simulink model "gm_CustArch_vnl"  (R2020a)
settings: Solver=FixedStepDiscrete  StartTime=0.0  StopTime=7e4  RelTol=1e-3
libraries: simulink x176, hdlsllib x104, hdlmdlgenlib x2, dsparch4 x1
(part 3 of 4)

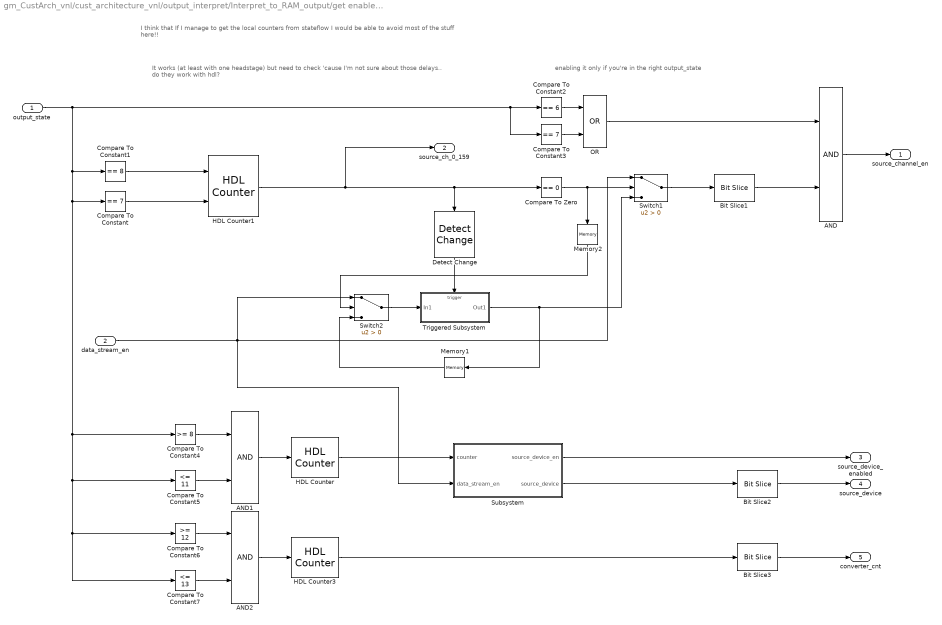
== system gm_CustArch_vnl/cust_architecture_vnl/output_interpret/Interpret_to_RAM_output/get enabled timings  ==
  note: It works (at least with one headstage) but need to check 'cause I'm not sure about those delays.. do they work with hdl?
  note: enabling it only if you're in the right output_state
  note: I think that If I manage to get the local counters from stateflow I would be able to avoid most of the stuff here!!
  output_state : Inport
  data_stream_en : Inport  Port=2
  AND : Logic  IconShape=distinctive  AllPortsSameDT=off  OutDataTypeStr=boolean
  AND1 : Logic  IconShape=distinctive  AllPortsSameDT=off  OutDataTypeStr=boolean
  AND2 : Logic  IconShape=distinctive  AllPortsSameDT=off  OutDataTypeStr=boolean
  Bit Slice1 : hdlsllib/Logic and Bit Operations/Bit Slice  lidx=0  ridx=0
      settings: SourceProductBaseCode=SL
  Bit Slice2 : hdlsllib/Logic and Bit Operations/Bit Slice  lidx=2  ridx=0
      settings: SourceProductBaseCode=SL
  Bit Slice3 : hdlsllib/Logic and Bit Operations/Bit Slice  lidx=2  ridx=0
      settings: SourceProductBaseCode=SL
  Compare To Constant : simulink/Logic and Bit Operations/Compare To Constant  relop===  const=7  OutDataTypeStr=boolean
  Compare To Constant1 : simulink/Logic and Bit Operations/Compare To Constant  relop===  const=8  OutDataTypeStr=boolean
  Compare To Constant2 : simulink/Logic and Bit Operations/Compare To Constant  relop===  const=6  OutDataTypeStr=boolean
  Compare To Constant3 : simulink/Logic and Bit Operations/Compare To Constant  relop===  const=7  OutDataTypeStr=boolean
  Compare To Constant4 : simulink/Logic and Bit Operations/Compare To Constant  relop=>=  const=8  OutDataTypeStr=boolean
  Compare To Constant5 : simulink/Logic and Bit Operations/Compare To Constant  relop=<=  const=11  OutDataTypeStr=boolean
  Compare To Constant6 : simulink/Logic and Bit Operations/Compare To Constant  relop=>=  const=12  OutDataTypeStr=boolean
  Compare To Constant7 : simulink/Logic and Bit Operations/Compare To Constant  relop=<=  const=13  OutDataTypeStr=boolean
  Compare To Zero : simulink/Logic and Bit Operations/Compare To Zero  relop===  OutDataTypeStr=boolean
  Detect Change : simulink/Logic and Bit Operations/Detect Change  vinit=0  OutDataTypeStr=boolean
  HDL Counter : hdlsllib/Sources/HDL Counter  CountType=Count limited  CountInit=0  CountStep=1  CountMax=7  CountFromType=Specify  CountFrom=0  CountResetPort=off  CountLoadPort=off  CountEnbPort=on  CountDirPort=off  CountDataType=Unsigned  CountWordLen=8  CountFracLen=0  CountSampTime=1
  HDL Counter1 : hdlsllib/Sources/HDL Counter  CountType=Count limited  CountInit=0  CountStep=1  CountMax=159  CountFromType=Specify  CountFrom=0  CountResetPort=on  CountLoadPort=off  CountEnbPort=on  CountDirPort=off  CountDataType=Unsigned  CountWordLen=8  CountFracLen=0  CountSampTime=1
  HDL Counter3 : hdlsllib/Sources/HDL Counter  CountType=Count limited  CountInit=0  CountStep=1  CountMax=7  CountFromType=Specify  CountFrom=0  CountResetPort=off  CountLoadPort=off  CountEnbPort=on  CountDirPort=off  CountDataType=Unsigned  CountWordLen=8  CountFracLen=0  CountSampTime=1
  Memory1 : Memory  InheritSampleTime=on
  Memory2 : Memory  InheritSampleTime=on
  OR : Logic  Operator=OR  IconShape=distinctive  AllPortsSameDT=off  OutDataTypeStr=boolean
  Subsystem : Subsystem
  Switch1 : Switch  Criteria=u2 > Threshold
  Switch2 : Switch  Criteria=u2 > Threshold
  Triggered Subsystem : Subsystem  TreatAsAtomicUnit=on
  source_channel_en : Outport  VectorParamsAs1DForOutWhenUnconnected=off
  source_ch_0_159 : Outport  Port=2  OutMin=0  OutMax=159  OutDataTypeStr=uint8  VectorParamsAs1DForOutWhenUnconnected=off  LockScale=on
  source_device_enabled : Outport  Port=3  VectorParamsAs1DForOutWhenUnconnected=off
  source_device : Outport  Port=4  VectorParamsAs1DForOutWhenUnconnected=off
  converter_cnt : Outport  Port=5  VectorParamsAs1DForOutWhenUnconnected=off
  wires:
  Compare To Constant/1 -> HDL Counter1/2
  Compare To Constant1/1 -> HDL Counter1/1
  HDL Counter3/1 -> Bit Slice3/1
  AND2/1 -> HDL Counter3/1
  Compare To Constant7/1 -> AND2/2
  output_state/1 -> Compare To Constant2/1, Compare To Constant3/1, Compare To Constant4/1, Compare To Constant5/1, Compare To Constant7/1, Compare To Constant6/1, Compare To Constant/1, Compare To Constant1/1
  Bit Slice3/1 -> converter_cnt/1
  Compare To Constant6/1 -> AND2/1
  data_stream_en/1 -> Switch2/1, Subsystem/2(data_stream_en), Switch1/1
  Subsystem/2(source_device) -> Bit Slice2/1
  HDL Counter/1 -> Subsystem/1("counter ")
  AND1/1 -> HDL Counter/1
  Bit Slice2/1 -> source_device/1
  Subsystem/1(source_device_en) -> source_device_enabled/1
  Compare To Constant5/1 -> AND1/2
  Compare To Constant4/1 -> AND1/1
  Bit Slice1/1 -> AND/2
  Switch1/1 -> Bit Slice1/1
  AND/1 -> source_channel_en/1
  OR/1 -> AND/1
  Compare To Constant2/1 -> OR/1
  Compare To Constant3/1 -> OR/2
  Memory2/1 -> Switch2/2
  Compare To Zero/1 -> Memory2/1, Switch1/2
  Switch2/1 -> Triggered Subsystem/1(In1)
  Memory1/1 -> Switch2/3
  Triggered Subsystem/1(Out1) -> Switch1/3, Memory1/1
  Detect Change/1 -> Triggered Subsystem/Trigger
  HDL Counter1/1 -> source_ch_0_159/1, Compare To Zero/1, Detect Change/1

== system gm_CustArch_vnl/cust_architecture_vnl/process_and_retrieve/80-120Hz IIR/Filter ==
  In : Inport
  Input Quantizer : DataTypeConversion  OutDataTypeStr=fixdt(1,16,15)  RndMeth=Round  SaturateOnIntegerOverflow=on
  filter : dsparch4/Biquad Filter  FilterSource=Dialog parameters  CoeffSource=Specify via dialog  FilterObject=BQF  IIRFiltStruct=Direct form II  BiQuadCoeffs=[1 0 -1 1 -1.99840418478311443 0.999052538203115237;1 0 -1 1 -1.99911154185162543 0.999384811657715533;1 0 -1 1 -1.99656292392472823 0.997202711747327109;1 0 -1 1 -1.99788402546849486 0.998160528507833211;1 0 -1 1 -1.99485713531997422 0.995480866402445264;1 0 -1 1 -1.99667039725885465 0.996953603258886489;1 0 -1 1 -1.99336016454168963 0.993961190148174412;1 0 -1 1 -1.99548437511557175 0.995777884172216132;1 0 -1 1 -1.992132714994862 0.992705563421812376;1 0 -1 1 -1.99434459502704264 0.994652174705462522;1 0 -1 1 -1.99121885243658769 0.991759490866001236;1 0 -1 1 -1.99327645890654415 0.99360203837599903;1 0 -1 1 -1.99064291385656711 0.991148910200749356;1 0 -1 1 -1.99231340829021986 0.992661008227186614;1 0 -1 1 -1.99040799304795324 0.990878552519449007;1 0 -1 1 -1.99149697231721445 0.991870551163973602;1 0 -1 1 -1.990496738771526 0.990932601430571158;1 0 -1 1 -1.99087486526267554 0.991278074310207646]  ScaleValues=[0.0044824738599215392;0.0044824738599215392;0.00447903005734254407;0.00447903005734254407;0.00447575140857445122;0.00447575140857445122;0.00447273615619287867;0.00447273615619287867;0.004470074082001705;0.004470074082001705;0.004467844000312143;0.004467844000312143;0.00446611161073571031;0.00446611161073571031;0.00446492774650666859;0.00446492774650666859;0.00446432704310449711;0.00446432704310449711;1]  IC=0  ICnum=0  ICden=0  a0Flag=Warning  optimizeScaleValues=on  ScaleValueMode=Specify via input port (g)  InputProcessing=Columns as channels (frame based)  roundingMode=Convergent  overflowMode=off  stageInputMode=Binary point scaling  stageInputWordLength=16  stageInputFracLength=17  stageOutputMode=Binary point scaling  stageOutputWordLength=16  stageOutputFracLength=11  firstCoeffMode=Binary point scaling  firstCoeffWordLength=16  firstCoeffFracLength=14  scaleValueFracLength=22  prodOutputMode=Binary point scaling  prodOutputWordLength=32  prodOutputFracLength=29  denProdOutputFracLength=29  accumMode=Binary point scaling  accumWordLength=40  accumFracLength=29  denAccumFracLength=29  memoryMode=Binary point scaling  memoryWordLength=16  memoryFracLength=15  secondMemoryFracLength=15  outputMode=Binary point scaling  outputWordLength=16  outputFracLength=11
  Out : Outport
  wires:
  filter/1 -> Out/1
  Input Quantizer/1 -> filter/1
  In/1 -> Input Quantizer/1

== system gm_CustArch_vnl/cust_architecture_vnl/process_and_retrieve/one_pole_IIR/Filter1 ==
  Input : Inport  OutDataTypeStr=fixdt(1,16,0)
  Input1 : Inport  Port=2
  SumA21 : Sum  Inputs=|+-  OutDataTypeStr=fixdt(1,16,-5)  RndMeth=Nearest  SaturateOnIntegerOverflow=on
  SumB21 : Sum  Inputs=|+-  OutDataTypeStr=fixdt(1,16,-1)  RndMeth=Nearest  SaturateOnIntegerOverflow=on
  a(2)(1) : Gain  Gain=-0.939062505817492399  ParamDataTypeStr=fixdt(1,16,15)  OutDataTypeStr=fixdt(1,16,-4)  RndMeth=Nearest  SaturateOnIntegerOverflow=on
  s(1) : Gain  Gain=0.969531252908746199  ParamDataTypeStr=fixdt(0,16,16)  OutDataTypeStr=fixdt(1,16,0)  RndMeth=Nearest  SaturateOnIntegerOverflow=on
  Output : Outport  VectorParamsAs1DForOutWhenUnconnected=off
  Output1 : Outport  Port=2  VectorParamsAs1DForOutWhenUnconnected=off
  wires:
  Input1/1 -> SumB21/2, a(2)(1)/1
  a(2)(1)/1 -> SumA21/2
  SumB21/1 -> Output/1
  SumA21/1 -> SumB21/1, Output1/1
  s(1)/1 -> SumA21/1
  Input/1 -> s(1)/1

== system gm_CustArch_vnl/cust_architecture/input_interpret_store_retrieve/Interpret_to_RAM_input/interpret data/condition to count DAC or ADC  ==
  fifo_write_to : Inport  OutDataTypeStr=boolean  PortDimensions=1  SampleTime=1
  input_state : Inport  Port=2  OutDataTypeStr=uint8  PortDimensions=1  SampleTime=1
  AND : Logic  AllPortsSameDT=off  OutDataTypeStr=boolean  SampleTime=1
  OR : Logic  Operator=OR  AllPortsSameDT=off  OutDataTypeStr=boolean  SampleTime=1
  is state_ADC : simulink/Logic and Bit Operations/Compare To Constant  relop===  const="fi(0,0,8,0,\"hex\",\"0d\")"  OutDataTypeStr=boolean
  is state_DAC : simulink/Logic and Bit Operations/Compare To Constant  relop===  const="fi(0,0,8,0,\"hex\",\"0c\")"  OutDataTypeStr=boolean
  Out1 : Outport  VectorParamsAs1DForOutWhenUnconnected=off
  wires:
  is state_DAC/1 -> OR/1
  is state_ADC/1 -> OR/2
  OR/1 -> AND/2
  AND/1 -> Out1/1
  input_state/1 -> is state_ADC/1, is state_DAC/1
  fifo_write_to/1 -> AND/1

== system gm_CustArch_vnl/cust_architecture/input_interpret_store_retrieve/Interpret_to_RAM_input/interpret data/get_sources ==
  note: 0-159 --> 20(16+4)x8
  note: chiedere cose
  note: identifichi chip che stai leggendo
  note: se next è tutto di zeri allora siamo a un nuovo channel (0-19)
  FIFO_write_to : Inport  OutDataTypeStr=boolean  PortDimensions=1  SampleTime=1
  InputState : Inport  Port=2  OutDataTypeStr=uint8  PortDimensions=1  SampleTime=1
  data_stream_enable : Inport  Port=3  OutDataTypeStr=uint8  PortDimensions=1  SampleTime=1
  AND{,1..3} (4 alike) : Logic  AllPortsSameDT=off  OutDataTypeStr=boolean  SampleTime=1
  Compare To Constant1 : simulink/Logic and Bit Operations/Compare To Constant  relop===  const="fi(0,0,8,0,\"hex\",\"00\")"  OutDataTypeStr=boolean
  Compare To Constant2 : simulink/Logic and Bit Operations/Compare To Constant  relop===  const="fi(0,0,8,0,\"hex\",\"0d\")"  OutDataTypeStr=boolean
  Compare To Constant3 : simulink/Logic and Bit Operations/Compare To Constant  relop===  const="fi(0,0,8,0,\"hex\",\"06\")"  OutDataTypeStr=boolean
  Compare To Constant4 : simulink/Logic and Bit Operations/Compare To Constant  relop=>=  const="fi(0,0,8,0,\"hex\",\"08\")"  OutDataTypeStr=boolean
  Compare To Constant5 : simulink/Logic and Bit Operations/Compare To Constant  relop===  const="fi(0,0,8,0,\"hex\",\"00\")"  OutDataTypeStr=boolean
  Compare To Constant6 : simulink/Logic and Bit Operations/Compare To Constant  relop=<=  const="fi(0,0,8,0,\"hex\",\"0b\")"  OutDataTypeStr=boolean
  HDL Counter : hdlsllib/Sources/HDL Counter  CountType=Count limited  CountInit=double(0)  CountStep=double(1)  CountMax=double(20)  CountFromType=Initial value  CountFrom=double(0)  CountResetPort=on  CountLoadPort=off  CountEnbPort=on  CountDirPort=off  CountDataType=Unsigned  CountWordLen=8  CountFracLen=0  CountSampTime=1
  Memory : UnitDelay  InitialCondition=double(0)  SampleTime=1
  Memory1 : UnitDelay  InitialCondition=double(0)  SampleTime=1
  Memory2 : UnitDelay  InitialCondition=double(0)  SampleTime=1
  OR : Logic  Operator=OR  AllPortsSameDT=off  OutDataTypeStr=boolean  SampleTime=1
  Subsystem : Subsystem
  Switch : Switch  Criteria=u2 > Threshold  Threshold=double(0)  OutDataTypeStr=uint8  SampleTime=1
  Switch1 : Switch  Criteria=u2 > Threshold  Threshold=double(0)  OutDataTypeStr=uint8  SampleTime=1
  Triggered Subsystem : Subsystem
  find_first_one_pos : Subsystem
  position_to_bitmask : Subsystem
  source_device : Outport  VectorParamsAs1DForOutWhenUnconnected=off
  dev_out_channel_0_19 : Outport  Port=2  VectorParamsAs1DForOutWhenUnconnected=off
  source_channel : Outport  Port=3  VectorParamsAs1DForOutWhenUnconnected=off
  bitmasked==0 : Outport  Port=4  VectorParamsAs1DForOutWhenUnconnected=off
  wires:
  position_to_bitmask/1(bit_masked) -> Memory/1, Compare To Constant5/1
  find_first_one_pos/1(first_one_pos) -> Triggered Subsystem/1(In1), position_to_bitmask/2(first_one_pos)
  Triggered Subsystem/1(Out1) -> Subsystem/1(source_device), source_device/1
  Switch1/1 -> Switch/3
  Switch/1 -> find_first_one_pos/1(In1), position_to_bitmask/1(curr_channel_rollmap)
  Subsystem/1(source_channel_0_159) -> source_channel/1
  OR/1 -> AND/2
  Memory2/1 -> AND3/2
  Memory1/1 -> AND3/1, Switch1/2
  Memory/1 -> Switch1/3
  HDL Counter/1 -> Subsystem/2(dev_output), dev_out_channel_0_19/1
  Compare To Constant6/1 -> AND1/2
  Compare To Constant5/1 -> Memory1/1, AND2/2
  Compare To Constant4/1 -> AND1/1
  Compare To Constant3/1 -> OR/1
  Compare To Constant2/1 -> HDL Counter/1
  Compare To Constant1/1 -> Switch/2
  AND3/1 -> HDL Counter/2
  AND2/1 -> bitmasked==0/1
  AND1/1 -> OR/2
  AND/1 -> find_first_one_pos/Enable, position_to_bitmask/Enable, Subsystem/Enable, Triggered Subsystem/Enable, Memory2/1, AND2/1
  data_stream_enable/1 -> Switch/1, Switch1/1
  InputState/1 -> Compare To Constant1/1, Compare To Constant2/1, Compare To Constant3/1, Compare To Constant4/1, Compare To Constant6/1
  FIFO_write_to/1 -> AND/1

== system gm_CustArch_vnl/cust_architecture/output_interpret/Interpret_to_RAM_output/get enabled timings /Subsystem ==
  "counter " : Inport  OutDataTypeStr=uint8  PortDimensions=1  SampleTime=1
  data_stream_en : Inport  Port=2  OutDataTypeStr=uint8  PortDimensions=1  SampleTime=1
  Bit Rotate : hdlsllib/Logic and Bit Operations/Bit Rotate  mode=Rotate Right  N=double(1)
      settings: SourceProductBaseCode=SL
  Bit Rotate1 : hdlsllib/Logic and Bit Operations/Bit Rotate  mode=Rotate Right  N=double(2)
      settings: SourceProductBaseCode=SL
  Bit Rotate2 : hdlsllib/Logic and Bit Operations/Bit Rotate  mode=Rotate Right  N=double(3)
      settings: SourceProductBaseCode=SL
  Bit Rotate3 : hdlsllib/Logic and Bit Operations/Bit Rotate  mode=Rotate Right  N=double(4)
      settings: SourceProductBaseCode=SL
  Bit Rotate4 : hdlsllib/Logic and Bit Operations/Bit Rotate  mode=Rotate Right  N=double(5)
      settings: SourceProductBaseCode=SL
  Bit Rotate5 : hdlsllib/Logic and Bit Operations/Bit Rotate  mode=Rotate Right  N=double(6)
      settings: SourceProductBaseCode=SL
  Bit Rotate6 : hdlsllib/Logic and Bit Operations/Bit Rotate  mode=Rotate Right  N=double(7)
      settings: SourceProductBaseCode=SL
  Bit Slice : hdlsllib/Logic and Bit Operations/Bit Slice  lidx=double(0)  ridx=double(0)
      settings: SourceProductBaseCode=SL
  Compare To Constant : simulink/Logic and Bit Operations/Compare To Constant  relop===  const="fi(0,0,8,0,\"hex\",\"00\")"  OutDataTypeStr=boolean
  Compare To Constant1 : simulink/Logic and Bit Operations/Compare To Constant  relop===  const="fi(0,0,8,0,\"hex\",\"01\")"  OutDataTypeStr=boolean
  Compare To Constant2 : simulink/Logic and Bit Operations/Compare To Constant  relop===  const="fi(0,0,8,0,\"hex\",\"02\")"  OutDataTypeStr=boolean
  Compare To Constant3 : simulink/Logic and Bit Operations/Compare To Constant  relop===  const="fi(0,0,8,0,\"hex\",\"03\")"  OutDataTypeStr=boolean
  Compare To Constant4 : simulink/Logic and Bit Operations/Compare To Constant  relop===  const="fi(0,0,8,0,\"hex\",\"04\")"  OutDataTypeStr=boolean
  Compare To Constant5 : simulink/Logic and Bit Operations/Compare To Constant  relop===  const="fi(0,0,8,0,\"hex\",\"05\")"  OutDataTypeStr=boolean
  Compare To Constant6 : simulink/Logic and Bit Operations/Compare To Constant  relop===  const="fi(0,0,8,0,\"hex\",\"06\")"  OutDataTypeStr=boolean
  Compare To Constant7 : simulink/Logic and Bit Operations/Compare To Constant  relop===  const="fi(0,0,8,0,\"hex\",\"07\")"  OutDataTypeStr=boolean
  Constant : Constant  Value=0  OutDataTypeStr=uint8  SampleTime=1
  Switch{,1..7} (8 alike) : Switch  Criteria=u2 > Threshold  Threshold=double(0)  OutDataTypeStr=uint8  SampleTime=1
  source_device_en : Outport  VectorParamsAs1DForOutWhenUnconnected=off
  source_device : Outport  Port=2  VectorParamsAs1DForOutWhenUnconnected=off
  wires:
  Switch7/1 -> Switch6/3
  Switch6/1 -> Switch5/3
  Switch5/1 -> Switch4/3
  Switch4/1 -> Switch3/3
  Switch3/1 -> Switch2/3
  Switch2/1 -> Switch1/3
  Switch1/1 -> Switch/3
  Switch/1 -> Bit Slice/1
  Constant/1 -> Switch7/3
  Compare To Constant7/1 -> Switch7/2
  Compare To Constant6/1 -> Switch6/2
  Compare To Constant5/1 -> Switch5/2
  Compare To Constant4/1 -> Switch4/2
  Compare To Constant3/1 -> Switch3/2
  Compare To Constant2/1 -> Switch2/2
  Compare To Constant1/1 -> Switch1/2
  Compare To Constant/1 -> Switch/2
  Bit Slice/1 -> source_device_en/1
  Bit Rotate6/1 -> Switch7/1
  Bit Rotate5/1 -> Switch6/1
  Bit Rotate4/1 -> Switch5/1
  Bit Rotate3/1 -> Switch4/1
  Bit Rotate2/1 -> Switch3/1
  Bit Rotate1/1 -> Switch2/1
  Bit Rotate/1 -> Switch1/1
  data_stream_en/1 -> Bit Rotate/1, Bit Rotate1/1, Bit Rotate2/1, Bit Rotate3/1, Bit Rotate4/1, Bit Rotate5/1, Bit Rotate6/1, Switch/1
  "counter "/1 -> source_device/1, Compare To Constant/1, Compare To Constant1/1, Compare To Constant2/1, Compare To Constant3/1, Compare To Constant4/1, Compare To Constant5/1, Compare To Constant6/1, Compare To Constant7/1

== system gm_CustArch_vnl/cust_architecture/output_interpret/Interpret_to_RAM_output/get enabled timings /Triggered Subsystem ==
  In1 : Inport  OutDataTypeStr=uint8  PortDimensions=1
  Trigger : TriggerPort  VariantControl=(inherit)  PortDimensions=1  OutDataTypeStr=boolean
  Bit Rotate : hdlsllib/Logic and Bit Operations/Bit Rotate  mode=Rotate Right  N=double(1)
      settings: SourceProductBaseCode=SL
  Out1 : Outport  InitialOutput=0  VectorParamsAs1DForOutWhenUnconnected=off
  wires:
  Bit Rotate/1 -> Out1/1
  In1/1 -> Bit Rotate/1

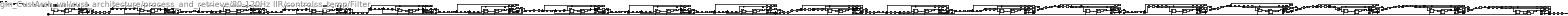
== system gm_CustArch_vnl/cust_architecture/process_and_retrieve/80-120Hz IIR/controlss_temp/Filter ==
  In : Inport  OutDataTypeStr=fixdt(1, 16, 15)  PortDimensions=1  SampleTime=1
  Trigger_emulated : Inport  Port=2  OutDataTypeStr=boolean  SampleTime=1
  Input Quantizer : DataTypeConversion  OutDataTypeStr=fixdt(1, 16, 15)  RndMeth=Round  SampleTime=1  SaturateOnIntegerOverflow=on
  Sub{,1..35} (36 alike) : Sum  Inputs=+-  OutDataTypeStr=fixdt(1, 41, 29)  RndMeth=Convergent  SampleTime=1
  adder{,1..17} (18 alike) : Sum  OutDataTypeStr=fixdt(1, 40, 29)  RndMeth=Convergent  SampleTime=1
  const : Constant  Value=0.0044825077056884765625  OutDataTypeStr=fixdt(1, 16, 22)  SampleTime=1
  const1 : Constant  Value=-1.9984130859375  OutDataTypeStr=fixdt(1, 16, 14)  SampleTime=1
  const10 : Constant  Value=-1.99786376953125  OutDataTypeStr=fixdt(1, 16, 14)  SampleTime=1
  const11 : Constant  Value=0.9981689453125  OutDataTypeStr=fixdt(1, 16, 14)  SampleTime=1
  const12 : Constant  Value=0.0044758319854736328125  OutDataTypeStr=fixdt(1, 16, 22)  SampleTime=1
  const13 : Constant  Value=-1.994873046875  OutDataTypeStr=fixdt(1, 16, 14)  SampleTime=1
  const14 : Constant  Value=0.9954833984375  OutDataTypeStr=fixdt(1, 16, 14)  SampleTime=1
  const15 : Constant  Value=0.0044758319854736328125  OutDataTypeStr=fixdt(1, 16, 22)  SampleTime=1
  const16 : Constant  Value=-1.99664306640625  OutDataTypeStr=fixdt(1, 16, 14)  SampleTime=1
  const17 : Constant  Value=0.9969482421875  OutDataTypeStr=fixdt(1, 16, 14)  SampleTime=1
  const18 : Constant  Value=0.0044727325439453125  OutDataTypeStr=fixdt(1, 16, 22)  SampleTime=1
  const19 : Constant  Value=-1.99334716796875  OutDataTypeStr=fixdt(1, 16, 14)  SampleTime=1
  const2 : Constant  Value=0.9990234375  OutDataTypeStr=fixdt(1, 16, 14)  SampleTime=1
  const20 : Constant  Value=0.99395751953125  OutDataTypeStr=fixdt(1, 16, 14)  SampleTime=1
  const21 : Constant  Value=0.0044727325439453125  OutDataTypeStr=fixdt(1, 16, 22)  SampleTime=1
  const22 : Constant  Value=-1.9954833984375  OutDataTypeStr=fixdt(1, 16, 14)  SampleTime=1
  const23 : Constant  Value=0.99578857421875  OutDataTypeStr=fixdt(1, 16, 14)  SampleTime=1
  const24 : Constant  Value=0.0044701099395751953125  OutDataTypeStr=fixdt(1, 16, 22)  SampleTime=1
  const25 : Constant  Value=-1.99212646484375  OutDataTypeStr=fixdt(1, 16, 14)  SampleTime=1
  const26 : Constant  Value=0.99267578125  OutDataTypeStr=fixdt(1, 16, 14)  SampleTime=1
  const27 : Constant  Value=0.0044701099395751953125  OutDataTypeStr=fixdt(1, 16, 22)  SampleTime=1
  const28 : Constant  Value=-1.99432373046875  OutDataTypeStr=fixdt(1, 16, 14)  SampleTime=1
  const29 : Constant  Value=0.99462890625  OutDataTypeStr=fixdt(1, 16, 14)  SampleTime=1
  const3 : Constant  Value=0.0044825077056884765625  OutDataTypeStr=fixdt(1, 16, 22)  SampleTime=1
  const30 : Constant  Value=0.0044677257537841796875  OutDataTypeStr=fixdt(1, 16, 22)  SampleTime=1
  const31 : Constant  Value=-1.9912109375  OutDataTypeStr=fixdt(1, 16, 14)  SampleTime=1
  const32 : Constant  Value=0.99176025390625  OutDataTypeStr=fixdt(1, 16, 14)  SampleTime=1
  const33 : Constant  Value=0.0044677257537841796875  OutDataTypeStr=fixdt(1, 16, 22)  SampleTime=1
  const34 : Constant  Value=-1.9932861328125  OutDataTypeStr=fixdt(1, 16, 14)  SampleTime=1
  const35 : Constant  Value=0.99359130859375  OutDataTypeStr=fixdt(1, 16, 14)  SampleTime=1
  const36 : Constant  Value=0.00446605682373046875  OutDataTypeStr=fixdt(1, 16, 22)  SampleTime=1
  const37 : Constant  Value=-1.99066162109375  OutDataTypeStr=fixdt(1, 16, 14)  SampleTime=1
  const38 : Constant  Value=0.99114990234375  OutDataTypeStr=fixdt(1, 16, 14)  SampleTime=1
  const39 : Constant  Value=0.00446605682373046875  OutDataTypeStr=fixdt(1, 16, 22)  SampleTime=1
  const4 : Constant  Value=-1.99908447265625  OutDataTypeStr=fixdt(1, 16, 14)  SampleTime=1
  const40 : Constant  Value=-1.9923095703125  OutDataTypeStr=fixdt(1, 16, 14)  SampleTime=1
  const41 : Constant  Value=0.99267578125  OutDataTypeStr=fixdt(1, 16, 14)  SampleTime=1
  const42 : Constant  Value=0.0044648647308349609375  OutDataTypeStr=fixdt(1, 16, 22)  SampleTime=1
  const43 : Constant  Value=-1.99041748046875  OutDataTypeStr=fixdt(1, 16, 14)  SampleTime=1
  const44 : Constant  Value=0.99090576171875  OutDataTypeStr=fixdt(1, 16, 14)  SampleTime=1
  const45 : Constant  Value=0.0044648647308349609375  OutDataTypeStr=fixdt(1, 16, 22)  SampleTime=1
  const46 : Constant  Value=-1.99151611328125  OutDataTypeStr=fixdt(1, 16, 14)  SampleTime=1
  const47 : Constant  Value=0.99188232421875  OutDataTypeStr=fixdt(1, 16, 14)  SampleTime=1
  const48 : Constant  Value=0.0044643878936767578125  OutDataTypeStr=fixdt(1, 16, 22)  SampleTime=1
  const49 : Constant  Value=-1.990478515625  OutDataTypeStr=fixdt(1, 16, 14)  SampleTime=1
  const5 : Constant  Value=0.9993896484375  OutDataTypeStr=fixdt(1, 16, 14)  SampleTime=1
  const50 : Constant  Value=0.99090576171875  OutDataTypeStr=fixdt(1, 16, 14)  SampleTime=1
  const51 : Constant  Value=0.0044643878936767578125  OutDataTypeStr=fixdt(1, 16, 22)  SampleTime=1
  const52 : Constant  Value=-1.9908447265625  OutDataTypeStr=fixdt(1, 16, 14)  SampleTime=1
  const53 : Constant  Value=0.99127197265625  OutDataTypeStr=fixdt(1, 16, 14)  SampleTime=1
  const6 : Constant  Value=0.004478931427001953125  OutDataTypeStr=fixdt(1, 16, 22)  SampleTime=1
  const7 : Constant  Value=-1.99658203125  OutDataTypeStr=fixdt(1, 16, 14)  SampleTime=1
  const8 : Constant  Value=0.9971923828125  OutDataTypeStr=fixdt(1, 16, 14)  SampleTime=1
  const9 : Constant  Value=0.004478931427001953125  OutDataTypeStr=fixdt(1, 16, 22)  SampleTime=1
  delay_process_section10_tap0 : Subsystem
      settings: MinAlgLoopOccurrences=on
  delay_process_section10_tap1 : Subsystem
      settings: MinAlgLoopOccurrences=on
  delay_process_section11_tap0 : Subsystem
      settings: MinAlgLoopOccurrences=on
  delay_process_section11_tap1 : Subsystem
      settings: MinAlgLoopOccurrences=on
  delay_process_section12_tap0 : Subsystem
      settings: MinAlgLoopOccurrences=on
  delay_process_section12_tap1 : Subsystem
      settings: MinAlgLoopOccurrences=on
  delay_process_section13_tap0 : Subsystem
      settings: MinAlgLoopOccurrences=on
  delay_process_section13_tap1 : Subsystem
      settings: MinAlgLoopOccurrences=on
  delay_process_section14_tap0 : Subsystem
      settings: MinAlgLoopOccurrences=on
  delay_process_section14_tap1 : Subsystem
      settings: MinAlgLoopOccurrences=on
  delay_process_section15_tap0 : Subsystem
      settings: MinAlgLoopOccurrences=on
  delay_process_section15_tap1 : Subsystem
      settings: MinAlgLoopOccurrences=on
  delay_process_section16_tap0 : Subsystem
      settings: MinAlgLoopOccurrences=on
  delay_process_section16_tap1 : Subsystem
      settings: MinAlgLoopOccurrences=on
  delay_process_section17_tap0 : Subsystem
      settings: MinAlgLoopOccurrences=on
  delay_process_section17_tap1 : Subsystem
      settings: MinAlgLoopOccurrences=on
  delay_process_section18_tap0 : Subsystem
      settings: MinAlgLoopOccurrences=on
  delay_process_section18_tap1 : Subsystem
      settings: MinAlgLoopOccurrences=on
  delay_process_section1_tap0 : Subsystem
      settings: MinAlgLoopOccurrences=on
  delay_process_section1_tap1 : Subsystem
      settings: MinAlgLoopOccurrences=on
  delay_process_section2_tap0 : Subsystem
      settings: MinAlgLoopOccurrences=on
  delay_process_section2_tap1 : Subsystem
      settings: MinAlgLoopOccurrences=on
  delay_process_section3_tap0 : Subsystem
      settings: MinAlgLoopOccurrences=on
  delay_process_section3_tap1 : Subsystem
      settings: MinAlgLoopOccurrences=on
  delay_process_section4_tap0 : Subsystem
      settings: MinAlgLoopOccurrences=on
  delay_process_section4_tap1 : Subsystem
      settings: MinAlgLoopOccurrences=on
  delay_process_section5_tap0 : Subsystem
      settings: MinAlgLoopOccurrences=on
  delay_process_section5_tap1 : Subsystem
      settings: MinAlgLoopOccurrences=on
  delay_process_section6_tap0 : Subsystem
      settings: MinAlgLoopOccurrences=on
  delay_process_section6_tap1 : Subsystem
      settings: MinAlgLoopOccurrences=on
  delay_process_section7_tap0 : Subsystem
      settings: MinAlgLoopOccurrences=on
  delay_process_section7_tap1 : Subsystem
      settings: MinAlgLoopOccurrences=on
  delay_process_section8_tap0 : Subsystem
      settings: MinAlgLoopOccurrences=on
  delay_process_section8_tap1 : Subsystem
      settings: MinAlgLoopOccurrences=on
  delay_process_section9_tap0 : Subsystem
      settings: MinAlgLoopOccurrences=on
  delay_process_section9_tap1 : Subsystem
      settings: MinAlgLoopOccurrences=on
  dtc{,11,22,33,44,55,66,77,88,99,110,121,132,143,154,165,176,187} (18 alike) : DataTypeConversion  OutDataTypeStr=fixdt(1, 16, 17)  RndMeth=Convergent  SampleTime=1
  dtc{1,12,23,34,45,56,67,78,89,100,111,122,133,144,155,166,177,188} (18 alike) : DataTypeConversion  OutDataTypeStr=fixdt(1, 16, 15)  RndMeth=Convergent  SampleTime=1
  dtc{10,21,32,43,54,65,76,87,98,109,120,131,142,153,164,175,186,197} (18 alike) : DataTypeConversion  OutDataTypeStr=fixdt(1, 16, 11)  RndMeth=Convergent  SampleTime=1
  dtc{2..9,13..20,24..31,35..42,46..53,57..64,68..75,79..86,90..97,101..108,112..119,123..130,134..141,145..152,156..163,167..174,178..185,189..196} (144 alike) : DataTypeConversion  OutDataTypeStr=fixdt(1, 40, 29)  RndMeth=Convergent  SampleTime=1
  filter_out1 : hdlmdlgenlib/Buffer
      settings: SourceProductBaseCode=SL
  gain{,2,4,6,8,10,12,14,16,18,20,22,24,26,28,30,32,34} (18 alike) : Gain  Gain="fi(0,1,16,14,\"hex\",\"4000\")"  ParamDataTypeStr=fixdt(1, 16, 14)  OutDataTypeStr=fixdt(1, 32, 29)  RndMeth=Convergent  SampleTime=1
  gain{1,3,5,7,9,11,13,15,17,19,21,23,25,27,29,31,33,35} (18 alike) : Gain  Gain="fi(0,1,16,14,\"hex\",\"c000\")"  ParamDataTypeStr=fixdt(1, 16, 14)  OutDataTypeStr=fixdt(1, 32, 29)  RndMeth=Convergent  SampleTime=1
  multiplier{,3,6,9,12,15,18,21,24,27,30,33,36,39,42,45,48,51} (18 alike) : Product  Inputs=**  OutDataTypeStr=fixdt(1, 36, 37)  RndMeth=Convergent  SampleTime=1
  multiplier{1..2,4..5,7..8,10..11,13..14,16..17,19..20,22..23,25..26,28..29,31..32,34..35,37..38,40..41,43..44,46..47,49..50,52..53} (36 alike) : Product  Inputs=**  OutDataTypeStr=fixdt(1, 32, 29)  RndMeth=Convergent  SampleTime=1
  output_typeconvert_wire : hdlmdlgenlib/Buffer
      settings: SourceProductBaseCode=SL
  t{,1..17} (18 alike) : Demux  Outputs=2
  t{18..35} (18 alike) : Mux  Inputs=2
  Out : Outport  InitialOutput=0
  wires:
  Trigger_emulated/1 -> delay_process_section1_tap0/Enable, delay_process_section1_tap1/Enable, delay_process_section2_tap0/Enable, delay_process_section2_tap1/Enable, delay_process_section3_tap0/Enable, delay_process_section3_tap1/Enable, delay_process_section4_tap0/Enable, delay_process_section4_tap1/Enable, delay_process_section5_tap0/Enable, delay_process_section5_tap1/Enable, delay_process_section6_tap0/Enable, delay_process_section6_tap1/Enable, delay_process_section7_tap0/Enable, delay_process_section7_tap1/Enable, delay_process_section8_tap0/Enable, delay_process_section8_tap1/Enable, delay_process_section9_tap0/Enable, delay_process_section9_tap1/Enable, delay_process_section10_tap0/Enable, delay_process_section10_tap1/Enable, delay_process_section11_tap0/Enable, delay_process_section11_tap1/Enable, delay_process_section12_tap0/Enable, delay_process_section12_tap1/Enable, delay_process_section13_tap0/Enable, delay_process_section13_tap1/Enable, delay_process_section14_tap0/Enable, delay_process_section14_tap1/Enable, delay_process_section15_tap0/Enable, delay_process_section15_tap1/Enable, delay_process_section16_tap0/Enable, delay_process_section16_tap1/Enable, delay_process_section17_tap0/Enable, delay_process_section17_tap1/Enable, delay_process_section18_tap0/Enable, delay_process_section18_tap1/Enable
  delay_process_section18_tap1/1(out0) -> t35/2
  delay_process_section18_tap0/1(out0) -> t35/1, delay_process_section18_tap1/1(in0)
  delay_process_section17_tap1/1(out0) -> t34/2
  delay_process_section17_tap0/1(out0) -> t34/1, delay_process_section17_tap1/1(in0)
  delay_process_section16_tap1/1(out0) -> t33/2
  delay_process_section16_tap0/1(out0) -> t33/1, delay_process_section16_tap1/1(in0)
  delay_process_section15_tap1/1(out0) -> t32/2
  delay_process_section15_tap0/1(out0) -> t32/1, delay_process_section15_tap1/1(in0)
  delay_process_section14_tap1/1(out0) -> t31/2
  delay_process_section14_tap0/1(out0) -> t31/1, delay_process_section14_tap1/1(in0)
  delay_process_section13_tap1/1(out0) -> t30/2
  delay_process_section13_tap0/1(out0) -> t30/1, delay_process_section13_tap1/1(in0)
  delay_process_section12_tap1/1(out0) -> t29/2
  delay_process_section12_tap0/1(out0) -> t29/1, delay_process_section12_tap1/1(in0)
  delay_process_section11_tap1/1(out0) -> t28/2
  delay_process_section11_tap0/1(out0) -> t28/1, delay_process_section11_tap1/1(in0)
  delay_process_section10_tap1/1(out0) -> t27/2
  delay_process_section10_tap0/1(out0) -> t27/1, delay_process_section10_tap1/1(in0)
  delay_process_section9_tap1/1(out0) -> t26/2
  delay_process_section9_tap0/1(out0) -> t26/1, delay_process_section9_tap1/1(in0)
  delay_process_section8_tap1/1(out0) -> t25/2
  delay_process_section8_tap0/1(out0) -> t25/1, delay_process_section8_tap1/1(in0)
  delay_process_section7_tap1/1(out0) -> t24/2
  delay_process_section7_tap0/1(out0) -> t24/1, delay_process_section7_tap1/1(in0)
  delay_process_section6_tap1/1(out0) -> t23/2
  delay_process_section6_tap0/1(out0) -> t23/1, delay_process_section6_tap1/1(in0)
  delay_process_section5_tap1/1(out0) -> t22/2
  delay_process_section5_tap0/1(out0) -> t22/1, delay_process_section5_tap1/1(in0)
  delay_process_section4_tap1/1(out0) -> t21/2
  delay_process_section4_tap0/1(out0) -> t21/1, delay_process_section4_tap1/1(in0)
  delay_process_section3_tap1/1(out0) -> t20/2
  delay_process_section3_tap0/1(out0) -> t20/1, delay_process_section3_tap1/1(in0)
  delay_process_section2_tap1/1(out0) -> t19/2
  delay_process_section2_tap0/1(out0) -> t19/1, delay_process_section2_tap1/1(in0)
  delay_process_section1_tap1/1(out0) -> t18/2
  delay_process_section1_tap0/1(out0) -> t18/1, delay_process_section1_tap1/1(in0)
  dtc197/1 -> output_typeconvert_wire/1
  dtc196/1 -> adder17/1
  Sub35/1 -> dtc195/1
  dtc194/1 -> Sub35/2
  dtc193/1 -> Sub35/1
  Sub34/1 -> dtc192/1
  dtc191/1 -> Sub34/2
  dtc190/1 -> Sub34/1
  gain35/1 -> adder17/2
  gain34/1 -> dtc196/1
  multiplier53/1 -> dtc194/1
  multiplier52/1 -> dtc191/1
  dtc189/1 -> dtc190/1
  t17/2 -> multiplier53/1, gain35/1
  t17/1 -> multiplier52/1
  t35/1 -> t17/1
  dtc188/1 -> gain34/1, delay_process_section18_tap0/1(in0)
  adder17/1 -> dtc197/1
  dtc192/1 -> dtc193/1
  dtc195/1 -> dtc188/1
  dtc187/1 -> dtc189/1
  const53/1 -> multiplier53/2
  const52/1 -> multiplier52/2
  multiplier51/1 -> dtc187/1
  const51/1 -> multiplier51/2
  dtc186/1 -> multiplier51/1
  dtc185/1 -> adder16/1
  Sub33/1 -> dtc184/1
  dtc183/1 -> Sub33/2
  dtc182/1 -> Sub33/1
  Sub32/1 -> dtc181/1
  dtc180/1 -> Sub32/2
  dtc179/1 -> Sub32/1
  gain33/1 -> adder16/2
  gain32/1 -> dtc185/1
  multiplier50/1 -> dtc183/1
  multiplier49/1 -> dtc180/1
  dtc178/1 -> dtc179/1
  t16/2 -> multiplier50/1, gain33/1
  t16/1 -> multiplier49/1
  t34/1 -> t16/1
  dtc177/1 -> gain32/1, delay_process_section17_tap0/1(in0)
  adder16/1 -> dtc186/1
  dtc181/1 -> dtc182/1
  dtc184/1 -> dtc177/1
  dtc176/1 -> dtc178/1
  const50/1 -> multiplier50/2
  const49/1 -> multiplier49/2
  multiplier48/1 -> dtc176/1
  const48/1 -> multiplier48/2
  dtc175/1 -> multiplier48/1
  dtc174/1 -> adder15/1
  Sub31/1 -> dtc173/1
  dtc172/1 -> Sub31/2
  dtc171/1 -> Sub31/1
  Sub30/1 -> dtc170/1
  dtc169/1 -> Sub30/2
  dtc168/1 -> Sub30/1
  gain31/1 -> adder15/2
  gain30/1 -> dtc174/1
  multiplier47/1 -> dtc172/1
  multiplier46/1 -> dtc169/1
  dtc167/1 -> dtc168/1
  t15/2 -> multiplier47/1, gain31/1
  t15/1 -> multiplier46/1
  t33/1 -> t15/1
  dtc166/1 -> gain30/1, delay_process_section16_tap0/1(in0)
  adder15/1 -> dtc175/1
  dtc170/1 -> dtc171/1
  dtc173/1 -> dtc166/1
  dtc165/1 -> dtc167/1
  const47/1 -> multiplier47/2
  const46/1 -> multiplier46/2
  multiplier45/1 -> dtc165/1
  const45/1 -> multiplier45/2
  dtc164/1 -> multiplier45/1
  dtc163/1 -> adder14/1
  Sub29/1 -> dtc162/1
  dtc161/1 -> Sub29/2
  dtc160/1 -> Sub29/1
  Sub28/1 -> dtc159/1
  dtc158/1 -> Sub28/2
  dtc157/1 -> Sub28/1
  gain29/1 -> adder14/2
  gain28/1 -> dtc163/1
  multiplier44/1 -> dtc161/1
  multiplier43/1 -> dtc158/1
  dtc156/1 -> dtc157/1
  t14/2 -> multiplier44/1, gain29/1
  t14/1 -> multiplier43/1
  t32/1 -> t14/1
  dtc155/1 -> gain28/1, delay_process_section15_tap0/1(in0)
  adder14/1 -> dtc164/1
  dtc159/1 -> dtc160/1
  dtc162/1 -> dtc155/1
  dtc154/1 -> dtc156/1
  const44/1 -> multiplier44/2
  const43/1 -> multiplier43/2
  multiplier42/1 -> dtc154/1
  const42/1 -> multiplier42/2
  dtc153/1 -> multiplier42/1
  dtc152/1 -> adder13/1
  Sub27/1 -> dtc151/1
  dtc150/1 -> Sub27/2
  dtc149/1 -> Sub27/1
  Sub26/1 -> dtc148/1
  dtc147/1 -> Sub26/2
  dtc146/1 -> Sub26/1
  gain27/1 -> adder13/2
  gain26/1 -> dtc152/1
  multiplier41/1 -> dtc150/1
  multiplier40/1 -> dtc147/1
  dtc145/1 -> dtc146/1
  t13/2 -> multiplier41/1, gain27/1
  t13/1 -> multiplier40/1
  t31/1 -> t13/1
  dtc144/1 -> gain26/1, delay_process_section14_tap0/1(in0)
  adder13/1 -> dtc153/1
  dtc148/1 -> dtc149/1
  dtc151/1 -> dtc144/1
  dtc143/1 -> dtc145/1
  const41/1 -> multiplier41/2
  const40/1 -> multiplier40/2
  multiplier39/1 -> dtc143/1
  const39/1 -> multiplier39/2
  dtc142/1 -> multiplier39/1
  dtc141/1 -> adder12/1
  Sub25/1 -> dtc140/1
  dtc139/1 -> Sub25/2
  dtc138/1 -> Sub25/1
  Sub24/1 -> dtc137/1
  dtc136/1 -> Sub24/2
  dtc135/1 -> Sub24/1
  gain25/1 -> adder12/2
  gain24/1 -> dtc141/1
  multiplier38/1 -> dtc139/1
  multiplier37/1 -> dtc136/1
  dtc134/1 -> dtc135/1
  t12/2 -> multiplier38/1, gain25/1
  t12/1 -> multiplier37/1
  t30/1 -> t12/1
  dtc133/1 -> gain24/1, delay_process_section13_tap0/1(in0)
  adder12/1 -> dtc142/1
  dtc137/1 -> dtc138/1
  dtc140/1 -> dtc133/1
  dtc132/1 -> dtc134/1
  const38/1 -> multiplier38/2
  const37/1 -> multiplier37/2
  multiplier36/1 -> dtc132/1
  const36/1 -> multiplier36/2
  dtc131/1 -> multiplier36/1
  dtc130/1 -> adder11/1
  Sub23/1 -> dtc129/1
  dtc128/1 -> Sub23/2
  dtc127/1 -> Sub23/1
  Sub22/1 -> dtc126/1
  dtc125/1 -> Sub22/2
  dtc124/1 -> Sub22/1
  gain23/1 -> adder11/2
  gain22/1 -> dtc130/1
  multiplier35/1 -> dtc128/1
  multiplier34/1 -> dtc125/1
  dtc123/1 -> dtc124/1
  t11/2 -> multiplier35/1, gain23/1
  t11/1 -> multiplier34/1
  t29/1 -> t11/1
  dtc122/1 -> gain22/1, delay_process_section12_tap0/1(in0)
  adder11/1 -> dtc131/1
  dtc126/1 -> dtc127/1
  dtc129/1 -> dtc122/1
  dtc121/1 -> dtc123/1
  const35/1 -> multiplier35/2
  const34/1 -> multiplier34/2
  multiplier33/1 -> dtc121/1
  const33/1 -> multiplier33/2
  dtc120/1 -> multiplier33/1
  dtc119/1 -> adder10/1
  Sub21/1 -> dtc118/1
  dtc117/1 -> Sub21/2
  dtc116/1 -> Sub21/1
  Sub20/1 -> dtc115/1
  dtc114/1 -> Sub20/2
  dtc113/1 -> Sub20/1
  gain21/1 -> adder10/2
  gain20/1 -> dtc119/1
  multiplier32/1 -> dtc117/1
  multiplier31/1 -> dtc114/1
  dtc112/1 -> dtc113/1
  t10/2 -> multiplier32/1, gain21/1
  t10/1 -> multiplier31/1
  t28/1 -> t10/1
  dtc111/1 -> gain20/1, delay_process_section11_tap0/1(in0)
  adder10/1 -> dtc120/1
  dtc115/1 -> dtc116/1
  dtc118/1 -> dtc111/1
  dtc110/1 -> dtc112/1
  const32/1 -> multiplier32/2
  const31/1 -> multiplier31/2
  multiplier30/1 -> dtc110/1
  const30/1 -> multiplier30/2
  dtc109/1 -> multiplier30/1
  dtc108/1 -> adder9/1
  Sub19/1 -> dtc107/1
  dtc106/1 -> Sub19/2
  dtc105/1 -> Sub19/1
  Sub18/1 -> dtc104/1
  dtc103/1 -> Sub18/2
  dtc102/1 -> Sub18/1
  gain19/1 -> adder9/2
  gain18/1 -> dtc108/1
  multiplier29/1 -> dtc106/1
  multiplier28/1 -> dtc103/1
  dtc101/1 -> dtc102/1
  t9/2 -> multiplier29/1, gain19/1
  t9/1 -> multiplier28/1
  t27/1 -> t9/1
  dtc100/1 -> gain18/1, delay_process_section10_tap0/1(in0)
  adder9/1 -> dtc109/1
  dtc104/1 -> dtc105/1
  dtc107/1 -> dtc100/1
  dtc99/1 -> dtc101/1
  const29/1 -> multiplier29/2
  const28/1 -> multiplier28/2
  multiplier27/1 -> dtc99/1
  const27/1 -> multiplier27/2
  dtc98/1 -> multiplier27/1
  dtc97/1 -> adder8/1
  Sub17/1 -> dtc96/1
  dtc95/1 -> Sub17/2
  dtc94/1 -> Sub17/1
  Sub16/1 -> dtc93/1
  dtc92/1 -> Sub16/2
  dtc91/1 -> Sub16/1
  gain17/1 -> adder8/2
  gain16/1 -> dtc97/1
  multiplier26/1 -> dtc95/1
  multiplier25/1 -> dtc92/1
  dtc90/1 -> dtc91/1
  t8/2 -> multiplier26/1, gain17/1
  t8/1 -> multiplier25/1
  t26/1 -> t8/1
  dtc89/1 -> gain16/1, delay_process_section9_tap0/1(in0)
  adder8/1 -> dtc98/1
  dtc93/1 -> dtc94/1
  dtc96/1 -> dtc89/1
  dtc88/1 -> dtc90/1
  const26/1 -> multiplier26/2
  const25/1 -> multiplier25/2
  multiplier24/1 -> dtc88/1
  const24/1 -> multiplier24/2
  dtc87/1 -> multiplier24/1
  dtc86/1 -> adder7/1
  Sub15/1 -> dtc85/1
  dtc84/1 -> Sub15/2
  dtc83/1 -> Sub15/1
  Sub14/1 -> dtc82/1
  dtc81/1 -> Sub14/2
  dtc80/1 -> Sub14/1
  gain15/1 -> adder7/2
  gain14/1 -> dtc86/1
  multiplier23/1 -> dtc84/1
  multiplier22/1 -> dtc81/1
  dtc79/1 -> dtc80/1
  t7/2 -> multiplier23/1, gain15/1
  t7/1 -> multiplier22/1
  t25/1 -> t7/1
  dtc78/1 -> gain14/1, delay_process_section8_tap0/1(in0)
  adder7/1 -> dtc87/1
  dtc82/1 -> dtc83/1
  dtc85/1 -> dtc78/1
  dtc77/1 -> dtc79/1
  const23/1 -> multiplier23/2
  const22/1 -> multiplier22/2
  multiplier21/1 -> dtc77/1
  const21/1 -> multiplier21/2
  dtc76/1 -> multiplier21/1
  dtc75/1 -> adder6/1
  Sub13/1 -> dtc74/1
  dtc73/1 -> Sub13/2
  dtc72/1 -> Sub13/1
  Sub12/1 -> dtc71/1
  dtc70/1 -> Sub12/2
  dtc69/1 -> Sub12/1
  gain13/1 -> adder6/2
  gain12/1 -> dtc75/1
  multiplier20/1 -> dtc73/1
  multiplier19/1 -> dtc70/1
  dtc68/1 -> dtc69/1
  t6/2 -> multiplier20/1, gain13/1
  t6/1 -> multiplier19/1
  t24/1 -> t6/1
  dtc67/1 -> gain12/1, delay_process_section7_tap0/1(in0)
  adder6/1 -> dtc76/1
  dtc71/1 -> dtc72/1
  dtc74/1 -> dtc67/1
  dtc66/1 -> dtc68/1
  const20/1 -> multiplier20/2
  const19/1 -> multiplier19/2
  multiplier18/1 -> dtc66/1
  const18/1 -> multiplier18/2
  dtc65/1 -> multiplier18/1
  dtc64/1 -> adder5/1
  Sub11/1 -> dtc63/1
  dtc62/1 -> Sub11/2
  dtc61/1 -> Sub11/1
  Sub10/1 -> dtc60/1
  dtc59/1 -> Sub10/2
  dtc58/1 -> Sub10/1
  gain11/1 -> adder5/2
  gain10/1 -> dtc64/1
  multiplier17/1 -> dtc62/1
  multiplier16/1 -> dtc59/1
  dtc57/1 -> dtc58/1
  t5/2 -> multiplier17/1, gain11/1
  t5/1 -> multiplier16/1
  t23/1 -> t5/1
  dtc56/1 -> gain10/1, delay_process_section6_tap0/1(in0)
  adder5/1 -> dtc65/1
  dtc60/1 -> dtc61/1
  dtc63/1 -> dtc56/1
  dtc55/1 -> dtc57/1
  const17/1 -> multiplier17/2
  const16/1 -> multiplier16/2
  multiplier15/1 -> dtc55/1
  const15/1 -> multiplier15/2
  dtc54/1 -> multiplier15/1
  dtc53/1 -> adder4/1
  Sub9/1 -> dtc52/1
  dtc51/1 -> Sub9/2
  dtc50/1 -> Sub9/1
  Sub8/1 -> dtc49/1
  dtc48/1 -> Sub8/2
  dtc47/1 -> Sub8/1
  gain9/1 -> adder4/2
  gain8/1 -> dtc53/1
  multiplier14/1 -> dtc51/1
  multiplier13/1 -> dtc48/1
  dtc46/1 -> dtc47/1
  t4/2 -> multiplier14/1, gain9/1
  t4/1 -> multiplier13/1
  t22/1 -> t4/1
  dtc45/1 -> gain8/1, delay_process_section5_tap0/1(in0)
  adder4/1 -> dtc54/1
  dtc49/1 -> dtc50/1
  dtc52/1 -> dtc45/1
  dtc44/1 -> dtc46/1
  const14/1 -> multiplier14/2
  const13/1 -> multiplier13/2
  multiplier12/1 -> dtc44/1
  const12/1 -> multiplier12/2
  dtc43/1 -> multiplier12/1
  dtc42/1 -> adder3/1
  Sub7/1 -> dtc41/1
  dtc40/1 -> Sub7/2
  dtc39/1 -> Sub7/1
  Sub6/1 -> dtc38/1
  dtc37/1 -> Sub6/2
  dtc36/1 -> Sub6/1
  gain7/1 -> adder3/2
  gain6/1 -> dtc42/1
  multiplier11/1 -> dtc40/1
  multiplier10/1 -> dtc37/1
  dtc35/1 -> dtc36/1
  t3/2 -> multiplier11/1, gain7/1
  t3/1 -> multiplier10/1
  t21/1 -> t3/1
  dtc34/1 -> gain6/1, delay_process_section4_tap0/1(in0)
  adder3/1 -> dtc43/1
  dtc38/1 -> dtc39/1
  dtc41/1 -> dtc34/1
  dtc33/1 -> dtc35/1
  const11/1 -> multiplier11/2
  const10/1 -> multiplier10/2
  multiplier9/1 -> dtc33/1
  const9/1 -> multiplier9/2
  dtc32/1 -> multiplier9/1
  dtc31/1 -> adder2/1
  Sub5/1 -> dtc30/1
  dtc29/1 -> Sub5/2
  dtc28/1 -> Sub5/1
  Sub4/1 -> dtc27/1
  dtc26/1 -> Sub4/2
  dtc25/1 -> Sub4/1
  gain5/1 -> adder2/2
  gain4/1 -> dtc31/1
  multiplier8/1 -> dtc29/1
  multiplier7/1 -> dtc26/1
  dtc24/1 -> dtc25/1
  t2/2 -> multiplier8/1, gain5/1
  t2/1 -> multiplier7/1
  t20/1 -> t2/1
  dtc23/1 -> gain4/1, delay_process_section3_tap0/1(in0)
  adder2/1 -> dtc32/1
  dtc27/1 -> dtc28/1
  dtc30/1 -> dtc23/1
  dtc22/1 -> dtc24/1
  const8/1 -> multiplier8/2
  const7/1 -> multiplier7/2
  multiplier6/1 -> dtc22/1
  const6/1 -> multiplier6/2
  dtc21/1 -> multiplier6/1
  dtc20/1 -> adder1/1
  Sub3/1 -> dtc19/1
  dtc18/1 -> Sub3/2
  dtc17/1 -> Sub3/1
  Sub2/1 -> dtc16/1
  dtc15/1 -> Sub2/2
  dtc14/1 -> Sub2/1
  gain3/1 -> adder1/2
  gain2/1 -> dtc20/1
  multiplier5/1 -> dtc18/1
  multiplier4/1 -> dtc15/1
  dtc13/1 -> dtc14/1
  t1/2 -> multiplier5/1, gain3/1
  t1/1 -> multiplier4/1
  t19/1 -> t1/1
  dtc12/1 -> gain2/1, delay_process_section2_tap0/1(in0)
  adder1/1 -> dtc21/1
  dtc16/1 -> dtc17/1
  dtc19/1 -> dtc12/1
  dtc11/1 -> dtc13/1
  const5/1 -> multiplier5/2
  const4/1 -> multiplier4/2
  multiplier3/1 -> dtc11/1
  const3/1 -> multiplier3/2
  dtc10/1 -> multiplier3/1
  dtc9/1 -> adder/1
  Sub1/1 -> dtc8/1
  dtc7/1 -> Sub1/2
  dtc6/1 -> Sub1/1
  Sub/1 -> dtc5/1
  dtc4/1 -> Sub/2
  dtc3/1 -> Sub/1
  gain1/1 -> adder/2
  gain/1 -> dtc9/1
  multiplier2/1 -> dtc7/1
  multiplier1/1 -> dtc4/1
  dtc2/1 -> dtc3/1
  t/2 -> multiplier2/1, gain1/1
  t/1 -> multiplier1/1
  t18/1 -> t/1
  dtc1/1 -> gain/1, delay_process_section1_tap0/1(in0)
  adder/1 -> dtc10/1
  dtc5/1 -> dtc6/1
  dtc8/1 -> dtc1/1
  dtc/1 -> dtc2/1
  const2/1 -> multiplier2/2
  const1/1 -> multiplier1/2
  multiplier/1 -> dtc/1
  const/1 -> multiplier/2
  output_typeconvert_wire/1 -> filter_out1/1
  filter_out1/1 -> Out/1
  Input Quantizer/1 -> multiplier/1
  In/1 -> Input Quantizer/1

== system gm_CustArch_vnl/cust_architecture_vnl/input_interpret_store_retrieve/Interpret_to_RAM_input/interpret data/condition to count DAC or ADC  ==
  fifo_write_to : Inport
  input_state : Inport  Port=2
  AND : Logic  IconShape=distinctive  AllPortsSameDT=off  OutDataTypeStr=boolean
  OR : Logic  Operator=OR  IconShape=distinctive  AllPortsSameDT=off  OutDataTypeStr=boolean
  is state_ADC : simulink/Logic and Bit Operations/Compare To Constant  relop===  const=13  OutDataTypeStr=boolean
  is state_DAC : simulink/Logic and Bit Operations/Compare To Constant  relop===  const=12  OutDataTypeStr=boolean
  Out1 : Outport  VectorParamsAs1DForOutWhenUnconnected=off
  wires:
  AND/1 -> Out1/1
  OR/1 -> AND/2
  fifo_write_to/1 -> AND/1
  is state_ADC/1 -> OR/2
  is state_DAC/1 -> OR/1
  input_state/1 -> is state_ADC/1, is state_DAC/1

== system gm_CustArch_vnl/cust_architecture_vnl/input_interpret_store_retrieve/Interpret_to_RAM_input/interpret data/get_sources ==
  note: se next è tutto di zeri allora siamo a un nuovo channel (0-19)
  note: identifichi chip che stai leggendo
  note: Perchè 6 e non 7?
      | perchè non mi frega
      | che sia AC o DC,
      | sto solo identificando
      | le sorgenti
  note: chiedere cose
  note: 0-159 --> 20(16+4)x8
  FIFO_write_to : Inport
  InputState : Inport  Port=2
  data_stream_enable : Inport  Port=3
  AND{,1..3} (4 alike) : Logic  IconShape=distinctive  AllPortsSameDT=off  OutDataTypeStr=boolean
  Compare To Constant1 : simulink/Logic and Bit Operations/Compare To Constant  relop===  const=0  OutDataTypeStr=boolean
  Compare To Constant2 : simulink/Logic and Bit Operations/Compare To Constant  relop===  const=13  OutDataTypeStr=boolean
  Compare To Constant3 : simulink/Logic and Bit Operations/Compare To Constant  relop===  const=6  OutDataTypeStr=boolean
  Compare To Constant4 : simulink/Logic and Bit Operations/Compare To Constant  relop=>=  const=8  OutDataTypeStr=boolean
  Compare To Constant5 : simulink/Logic and Bit Operations/Compare To Constant  relop===  const=0  OutDataTypeStr=boolean
  Compare To Constant6 : simulink/Logic and Bit Operations/Compare To Constant  relop=<=  const=11  OutDataTypeStr=boolean
  HDL Counter : hdlsllib/Sources/HDL Counter  CountType=Count limited  CountInit=0  CountStep=1  CountMax=20  CountFromType=Specify  CountFrom=0  CountResetPort=on  CountLoadPort=off  CountEnbPort=on  CountDirPort=off  CountDataType=Unsigned  CountWordLen=8  CountFracLen=0  CountSampTime=1
  Memory : Memory  InheritSampleTime=on
  Memory1 : Memory  InheritSampleTime=on
  Memory2 : Memory  InheritSampleTime=on
  OR : Logic  Operator=OR  IconShape=distinctive  AllPortsSameDT=off  OutDataTypeStr=boolean
  Subsystem : Subsystem
  Switch : Switch  Criteria=u2 > Threshold  OutDataTypeStr=uint8
  Switch1 : Switch  Criteria=u2 > Threshold
  Triggered Subsystem : Subsystem  TreatAsAtomicUnit=on
  find_first_one_pos : Subsystem
  position_to_bitmask : Subsystem
  source_device : Outport  VectorParamsAs1DForOutWhenUnconnected=off
  dev_out_channel_0_19 : Outport  Port=2  VectorParamsAs1DForOutWhenUnconnected=off
  source_channel : Outport  Port=3  VectorParamsAs1DForOutWhenUnconnected=off
  bitmasked==0 : Outport  Port=4  VectorParamsAs1DForOutWhenUnconnected=off
  wires:
  AND2/1 -> bitmasked==0/1
  Memory1/1 -> Switch1/2, AND3/1
  OR/1 -> AND/2
  AND1/1 -> OR/2
  Compare To Constant6/1 -> AND1/2
  Compare To Constant4/1 -> AND1/1
  Compare To Constant2/1 -> HDL Counter/1
  Subsystem/1(source_channel_0_159) -> source_channel/1  "source_channel_0_159"
  Compare To Constant3/1 -> OR/1
  Triggered Subsystem/1(Out1) -> Subsystem/1(source_device), source_device/1  "source_device"
  Memory2/1 -> AND3/2
  Memory/1 -> Switch1/3
  AND3/1 -> HDL Counter/2
  HDL Counter/1 -> Subsystem/2(dev_output), dev_out_channel_0_19/1  "dev_output"
  Compare To Constant5/1 -> Memory1/1, AND2/2
  Switch1/1 -> Switch/3
  AND/1 -> AND2/1, Memory2/1, find_first_one_pos/Enable, position_to_bitmask/Enable, Subsystem/Enable, Triggered Subsystem/Enable
  FIFO_write_to/1 -> AND/1
  position_to_bitmask/1(bit_masked) -> Compare To Constant5/1, Memory/1  "next_chann_rollmap"
  data_stream_enable/1 -> Switch/1, Switch1/1
  Compare To Constant1/1 -> Switch/2
  Switch/1 -> find_first_one_pos/1(In1), position_to_bitmask/1(curr_channel_rollmap)  "curr_channel_rollmap"
  InputState/1 -> Compare To Constant3/1, Compare To Constant4/1, Compare To Constant6/1, Compare To Constant2/1, Compare To Constant1/1  "input state"
  find_first_one_pos/1(first_one_pos) -> Triggered Subsystem/1(In1), position_to_bitmask/2(first_one_pos)  "source_device"
